simulink model "GOSH"  (Simulink 7.9)
settings: Solver=ode45  StartTime=0.0  StopTime=10.0  RelTol=1e-3
libraries: simulink x1
settings Model: Creator=Mihail  LastModifiedBy=Mihail

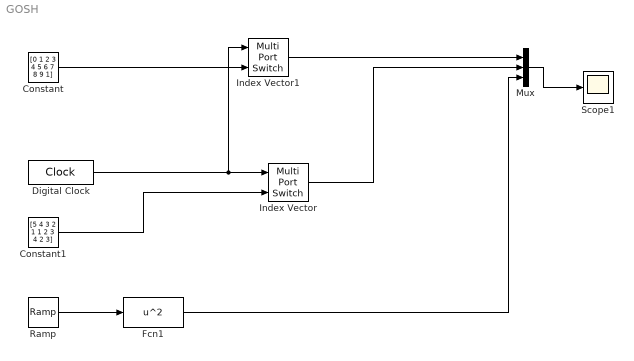
== system GOSH ==
  Constant : Constant  Value=[0 1 2 3 4 5 6 7 8 9 1]
  Constant1 : Constant  Value=[5 4 3 2 1 1 2 3 4 2 3]
  Digital Clock : DigitalClock
  Fcn1 : Fcn  Expr=u^2
  Index Vector : MultiPortSwitch  DataPortOrder=Zero-based contiguous  Inputs=1  zeroidx=on
  Index Vector1 : MultiPortSwitch  DataPortOrder=Zero-based contiguous  Inputs=1  zeroidx=on
  Mux : Mux  Inputs=3
  Ramp : simulink/Sources/Ramp  slope=1  start=0  X0=0
  Scope1 : Scope
      settings: TimeRange=0.06668296375670701  YMin=2.961430172622083  YMax=3.275129869258235
  wires:
  Constant1/1 -> Index Vector/2
  Constant/1 -> Index Vector1/2
  Index Vector1/1 -> Mux/1
  Index Vector/1 -> Mux/2
  Ramp/1 -> Fcn1/1
  Fcn1/1 -> Mux/3
  Digital Clock/1 -> Index Vector1/1, Index Vector/1
  Mux/1 -> Scope1/1
